simulink model "Leader_Follower_Simulation"  (R2015b)
settings: Solver=ode1  StartTime=0.0  StopTime=inf  FixedStep=0.001  RelTol=1e-3
libraries: simulink x1
settings Model: ExtModeTrigDuration=10000  Creator=ale  LastModifiedBy=anle
settings SolverCC: PositivePriorityOrder=on
settings RTWCC: SystemTargetFile=quarc_linux_duovero.tlc  TemplateMakefile=quarc_linux_duovero_tmf  Description=QUARC Linux DuoVero Target (QBall 2, QBot 2)
settings STFCustomTargetCC: TargetLibSuffix=.a  TargetPreCompLibLocation=C:\PROGRA~3\QUARC\lib\2015b\LINUX_~1\release  GeneratePreprocessorConditionals=Use local settings  CPPClassGenCompliant=off  SystemTargetFile=quarc_linux_duovero.tlc
settings GRTTargetCC: TargetLibSuffix=.a  TargetPreCompLibLocation=C:\PROGRA~3\QUARC\lib\2015b\LINUX_~1\release  ParMdlRefBuildCompliant=off  CompOptLevelCompliant=off  CombineOutputUpdateFcns=off  MatFileLogging=off  CPPClassGenCompliant=off  GRTInterface=on  UseToolchainInfoCompliant=off  ExtMode=on  ExtModeMexFile=quarc_comm  ExtModeMexArgs='-w -d /tmp -uri %u'

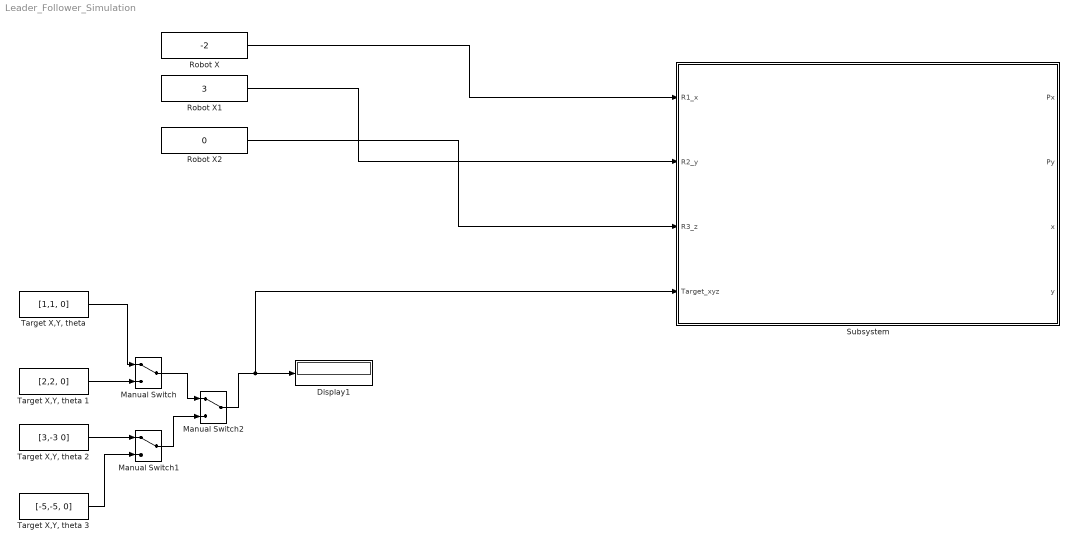
== system Leader_Follower_Simulation ==
  Display1 : Display
  Manual Switch : ManualSwitch
  Manual Switch1 : ManualSwitch
  Manual Switch2 : ManualSwitch
  Robot X : Constant  Value=-2
  Robot X1 : Constant  Value=3
  Robot X2 : Constant  Value=0
  Subsystem : Subsystem
  "Target X,Y, theta " : Constant  Value=[1,1, 0]
  "Target X,Y, theta 1" : Constant  Value=[2,2, 0]
  "Target X,Y, theta 2" : Constant  Value=[3,-3 0]
  "Target X,Y, theta 3" : Constant  Value=[-5,-5, 0]
  wires:
  Manual Switch2/1 -> Subsystem/4(Target_xyz), Display1/1
  "Target X,Y, theta "/1 -> Manual Switch/1
  "Target X,Y, theta 1"/1 -> Manual Switch/2
  Manual Switch/1 -> Manual Switch2/1
  Manual Switch1/1 -> Manual Switch2/2
  "Target X,Y, theta 2"/1 -> Manual Switch1/1
  "Target X,Y, theta 3"/1 -> Manual Switch1/2
  Robot X/1 -> Subsystem/1(R1_x)
  Robot X1/1 -> Subsystem/2(R2_y)
  Robot X2/1 -> Subsystem/3(R3_z)

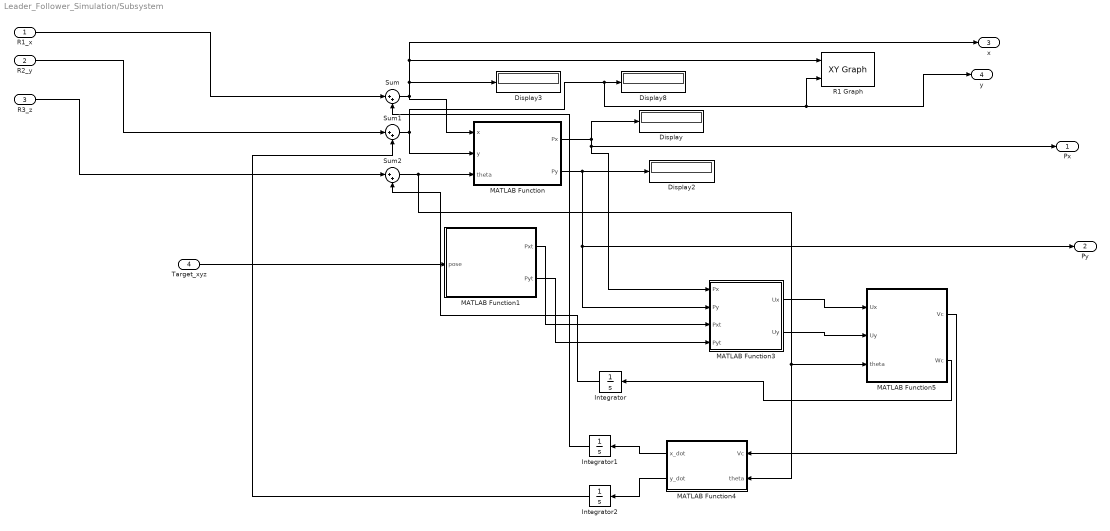
== system Leader_Follower_Simulation/Subsystem ==
  R1_x : Inport
  R2_y : Inport  Port=2
  R3_z : Inport  Port=3
  Target_xyz : Inport  Port=4
  Display{,2..3,8} (4 alike) : Display
  Integrator : Integrator
  Integrator1 : Integrator
  Integrator2 : Integrator
  MATLAB Function : MATLAB Function  TreatAsAtomicUnit=on
  MATLAB Function1 : MATLAB Function  TreatAsAtomicUnit=on
  MATLAB Function3 : MATLAB Function  TreatAsAtomicUnit=on
  MATLAB Function4 : MATLAB Function  TreatAsAtomicUnit=on
  MATLAB Function5 : MATLAB Function  TreatAsAtomicUnit=on
  R1 Graph : simulink/Sinks/XY Graph  xmin=-20  xmax=20  ymin=-20  ymax=20  st=-1
  Sum : Sum  Inputs=|++
  Sum1 : Sum  Inputs=|++
  Sum2 : Sum  Inputs=|++
  Px : Outport
  Py : Outport  Port=2
  x : Outport  Port=3
  y : Outport  Port=4
  wires:
  MATLAB Function1/1(Pxt) -> MATLAB Function3/3(Pxt)
  MATLAB Function1/2(Pyt) -> MATLAB Function3/4(Pyt)
  MATLAB Function/2(Py) -> Py/1, MATLAB Function3/2(Py), Display2/1
  MATLAB Function/1(Px) -> MATLAB Function3/1(Px), Px/1, Display/1
  Sum2/1 -> MATLAB Function4/2(theta), MATLAB Function5/3(theta), MATLAB Function/3(theta)
  Sum1/1 -> MATLAB Function/2(y), y/1, R1 Graph/2, Display8/1
  Sum/1 -> MATLAB Function/1(x), x/1, R1 Graph/1, Display3/1
  Target_xyz/1 -> MATLAB Function1/1(pose)
  MATLAB Function3/1(Ux) -> MATLAB Function5/1(Ux)
  MATLAB Function3/2(Uy) -> MATLAB Function5/2(Uy)
  MATLAB Function5/1(Vc) -> MATLAB Function4/1(Vc)
  MATLAB Function5/2(Wc) -> Integrator/1
  Integrator/1 -> Sum2/2
  MATLAB Function4/1(x_dot) -> Integrator1/1
  Integrator1/1 -> Sum/2
  MATLAB Function4/2(y_dot) -> Integrator2/1
  Integrator2/1 -> Sum1/2
  R1_x/1 -> Sum/1
  R2_y/1 -> Sum1/1
  R3_z/1 -> Sum2/1

== matlab function Leader_Follower_Simulation/Subsystem/MATLAB Function ==
  data: x input; Px output; Py output; y input; theta input
function [Px,Py] = PxPy_convert(x, y, theta)

l=.0235; %#length between the two wheels in meters
%R=.0175; %#R or signed distance from ICC (Instanteous center of curvature) in meters
Px= x+l*cos(theta)
Py = y+l*sin(theta)

%#codegen

== matlab function Leader_Follower_Simulation/Subsystem/MATLAB Function1 ==
  data: pose input; Pxt output; Pyt output
function [Pxt,Pyt] = PxtPyt_convert(pose)
x=pose(1);
y=pose(2);
theta=pose(2);
l=.0235; %#length between the two wheels in meters
%R=.0175; %#R or signed distance from ICC (Instanteous center of curvature) in meters
Pxt= x+l*cos(theta)
Pyt = y+l*sin(theta)

%#codegen

== matlab function Leader_Follower_Simulation/Subsystem/MATLAB Function3 ==
  data: Px input; Ux output; Py input; Pxt input; Pyt input; Uy output
function [Ux, Uy] = UxUy(Px,Py,Pxt,Pyt)
%#codegen
%rho_star=.5;
%omega_star=.5;
 
k = 0.2;

Ux = k*(Pxt-Px-.4);
Uy = k*(Pyt-Py-.4);

== matlab function Leader_Follower_Simulation/Subsystem/MATLAB Function4 ==
  data: Vc input; x_dot output; theta input; y_dot output
function [x_dot, y_dot] = VcWc2XYdot(Vc, theta)
%#codegen
x_dot = Vc*cos(theta)
y_dot = Vc*sin(theta)

== matlab function Leader_Follower_Simulation/Subsystem/MATLAB Function5 ==
  data: Ux input; Vc output; Uy input; Wc output; theta input
function [Vc,Wc] = UxUy2VcWc(Ux,Uy, theta)

l=.0235; %#length between the two wheels in meters
kin_inv = inv([cos(theta) -l*sin(theta) ; sin(theta) l*cos(theta)]);
P =  kin_inv*[Ux;Uy];
Vc=P(1);
Wc=P(2);
